simulink model "Observer_reduced_model"  (R2016b)
settings: Solver=ode45  StartTime=0.0  StopTime=1  FixedStep=0.0001  RelTol=1e-3
settings Model: Creator=emilio  LastModifiedBy=danielesmn

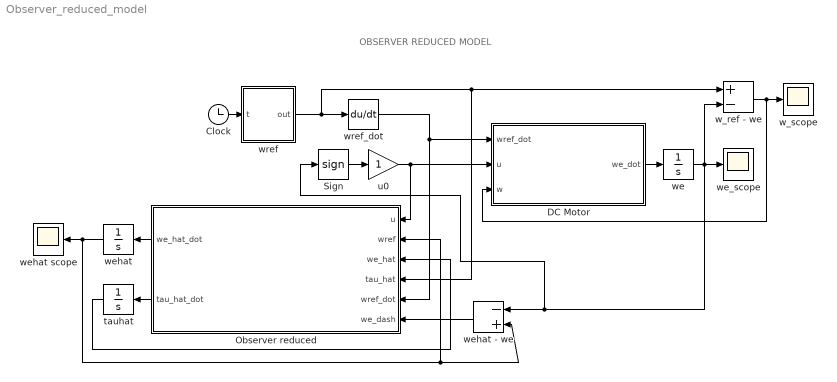
== system Observer_reduced_model ==
  note: OBSERVER REDUCED MODEL
  Clock : Clock
  DC Motor : MATLAB Function  TreatAsAtomicUnit=on
  "Observer reduced " : MATLAB Function  TreatAsAtomicUnit=on
  Sign : Signum  ZeroCross=off
  tauhat : Integrator
  u0 : Gain
  w_ref - we : Sum  Inputs=+-
  w_scope : Scope
  we : Integrator
  we_scope : Scope
  wehat : Integrator
  wehat - we : Sum  Inputs=-+
  wehat scope : Scope
  wref : MATLAB Function  TreatAsAtomicUnit=on
  wref_dot : Derivative
  wires:
  DC Motor/1(we_dot) -> we/1
  we/1 -> Sign/1, wehat - we/1, we_scope/1, w_ref - we/2
  wref_dot/1 -> DC Motor/1(wref_dot), "Observer reduced "/5(wref_dot)
  w_ref - we/1 -> DC Motor/3(w), w_scope/1
  Sign/1 -> u0/1
  u0/1 -> DC Motor/2(u), "Observer reduced "/1(u)
  Clock/1 -> wref/1(t)
  wref/1(out) -> "Observer reduced "/4(tau_hat), w_ref - we/1, wref_dot/1
  "Observer reduced "/2(tau_hat_dot) -> tauhat/1
  "Observer reduced "/1(we_hat_dot) -> wehat/1
  wehat/1 -> wehat - we/2, "Observer reduced "/2(wref), wehat scope/1
  wehat - we/1 -> "Observer reduced "/6(we_dash)
  tauhat/1 -> "Observer reduced "/3(we_hat)

== matlab function Observer_reduced_model/DC Motor ==
  data: wref_dot input; u input; we_dot output; w input
function we_dot = DC_Motor(wref_dot, u, w)

R = 0.5;          %Armature resistance (Ohm)
kt = 0.008;       %Torque constant (Nm/A)
J = 0.001;        %Inertia of the motor rotor (Kg*m^2)
B = 0.01;         %Coefficient of viscous friction (Nm*s/rad)
lambda0 = 0.001;  %Back electromotive force (EMF) constant (V*s/rad)
tau = B*w;

we_dot = kt*lambda0/(J*R)*w - kt/(J*R)*u + tau/J + wref_dot;

== matlab function Observer_reduced_model/Observer reduced  ==
  data: u input; we_hat_dot output; wref input; we_hat input; tau_hat input; wref_dot input; we_dash input; tau_hat_dot output
function  [we_hat_dot, tau_hat_dot] = ObsReduced(u, wref, we_hat, tau_hat, wref_dot, we_dash)

R = 0.5;          %Armature resistance (Ohm)
kt = 0.008;       %Torque constant (Nm/A)
J = 0.001;        %Inertia of the motor rotor (Kg*m^2)
B = 0.01;         %Coefficient of viscous friction (Nm*s/rad)
lambda0 = 0.001;  %Back electromotive force (EMF) constant (V*s/rad)

l1 = 20;          %Observer gain 1
l2 = 20;          %Observer gain 2

we_hat_dot = kt*lambda0/(J*R)*(wref - we_hat) - kt/(J*R)*u + tau_hat/J + wref_dot - l1/J*we_dash;
tau_hat_dot = -l2*we_dash;

== matlab function Observer_reduced_model/wref ==
  data: t input; out output
function out = input(t)

if t < 0.5
    out = 1;
else
    out = -1;
end
